simulink model "model"  (R2012b)
settings: Solver=ode45  StartTime=0.0  StopTime=10.0  MaxStep=0.2  RelTol=1e-3
settings Model: Creator=Vojta  LastModifiedBy=Pavilion
settings DataIOCC: SignalLoggingSaveFormat=ModelDataLogs
settings OptimizationCC: ExpressionDepthLimit=128
settings DebuggingCC: MultiTaskDSMMsg=warning  MultiTaskCondExecSysMsg=none  StateNameClashWarn=none  StrictBusMsg=None
settings RTWCC: IncludeERTFirstTime=on
settings CodeAppCC: CustomSymbolStrType=$N$R$M_T  InternalIdentifier=Shortened

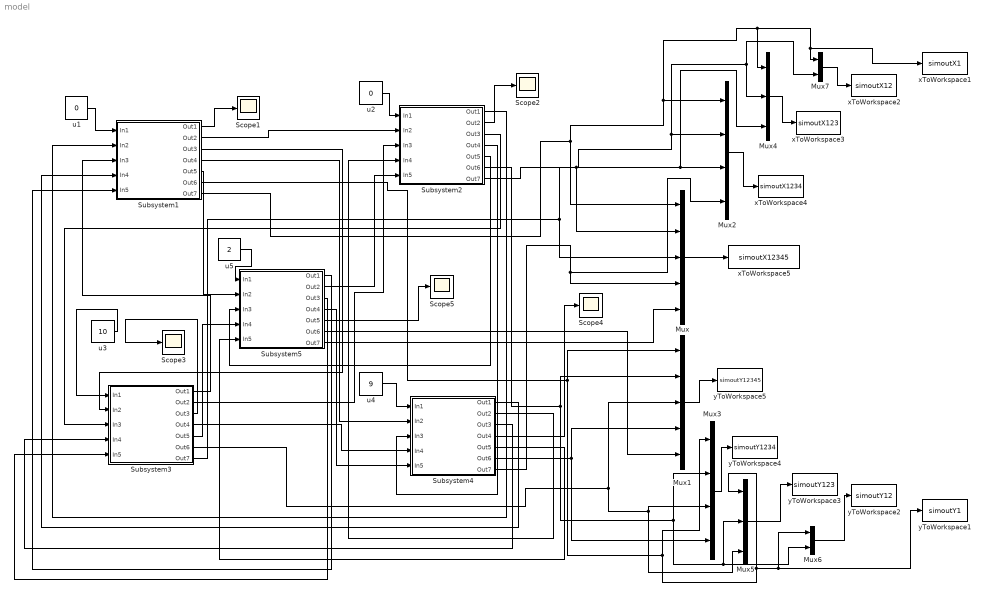
== system model ==
  Mux : Mux  Inputs=5
  Mux1 : Mux  Inputs=5
  Mux2 : Mux
  Mux3 : Mux
  Mux4 : Mux  Inputs=3
  Mux5 : Mux  Inputs=3
  Mux6 : Mux  Inputs=2
  Mux7 : Mux  Inputs=2
  Scope{1..5} (5 alike) : Scope
      Scope2 settings: SaveName=ScopeData2
      Scope3 settings: SaveName=ScopeData3
      Scope4 settings: SaveName=ScopeData4
      Scope5 settings: SaveName=ScopeData5
  Subsystem1 : Subsystem
  Subsystem2 : Subsystem
  Subsystem3 : Subsystem
  Subsystem4 : Subsystem
  Subsystem5 : Subsystem
  u1 : Constant  Value=0
  u2 : Constant  Value=0
  u3 : Constant  Value=10
  u4 : Constant  Value=9
  u5 : Constant  Value=2
  xToWorkspace1 : ToWorkspace  VariableName=simoutX1  SampleTime=-1  SaveFormat=Timeseries
  xToWorkspace2 : ToWorkspace  VariableName=simoutX12  SampleTime=-1  SaveFormat=Structure With Time
  xToWorkspace3 : ToWorkspace  VariableName=simoutX123  SampleTime=-1  SaveFormat=Structure With Time
  xToWorkspace4 : ToWorkspace  VariableName=simoutX1234  SampleTime=-1  SaveFormat=Structure With Time
  xToWorkspace5 : ToWorkspace  VariableName=simoutX12345  SampleTime=-1  SaveFormat=Structure With Time
  yToWorkspace1 : ToWorkspace  VariableName=simoutY1  SampleTime=-1  SaveFormat=Timeseries
  yToWorkspace2 : ToWorkspace  VariableName=simoutY12  SampleTime=-1  SaveFormat=Structure With Time
  yToWorkspace3 : ToWorkspace  VariableName=simoutY123  SampleTime=-1  SaveFormat=Structure With Time
  yToWorkspace4 : ToWorkspace  VariableName=simoutY1234  SampleTime=-1  SaveFormat=Structure With Time
  yToWorkspace5 : ToWorkspace  VariableName=simoutY12345  SampleTime=-1  SaveFormat=Structure With Time
  wires:
  u1/1 -> Subsystem1/1(In1)
  u2/1 -> Subsystem2/1(In1)
  u3/1 -> Subsystem3/1(In1)
  u4/1 -> Subsystem4/1(In1)
  u5/1 -> Subsystem5/1(In1)
  Subsystem1/7(Out7) -> xToWorkspace1/1, Mux7/1, Mux4/1, Mux2/1, Mux/1
  Subsystem2/7(Out7) -> Mux7/2, Mux4/2, Mux2/2, Mux/2
  Subsystem3/7(Out7) -> Mux4/3, Mux2/3, Mux/3
  Subsystem4/7(Out7) -> Mux/4, Mux2/4
  Subsystem1/6(Out6) -> yToWorkspace1/1, Mux6/1, Mux5/1, Mux3/1, Mux1/1
  Subsystem2/6(Out6) -> Mux6/2, Mux5/2, Mux3/2, Mux1/2
  Subsystem4/6(Out6) -> Mux3/4, Mux1/4
  Subsystem3/6(Out6) -> Mux1/3, Mux5/3, Mux3/3
  Mux/1 -> xToWorkspace5/1
  Mux1/1 -> yToWorkspace5/1
  Subsystem1/2(Out2) -> Subsystem2/2(In2)
  Subsystem1/3(Out3) -> Subsystem3/2(In2)
  Subsystem1/4(Out4) -> Subsystem4/2(In2)
  Subsystem1/5(Out5) -> Subsystem5/2(In2)
  Subsystem2/1(Out1) -> Subsystem1/2(In2)
  Subsystem2/3(Out3) -> Subsystem3/3(In3)
  Subsystem2/4(Out4) -> Subsystem4/3(In3)
  Subsystem2/5(Out5) -> Subsystem5/3(In3)
  Subsystem3/1(Out1) -> Subsystem1/3(In3)
  Subsystem3/2(Out2) -> Subsystem2/3(In3)
  Subsystem3/4(Out4) -> Subsystem4/4(In4)
  Subsystem3/5(Out5) -> Subsystem5/4(In4)
  Subsystem4/1(Out1) -> Subsystem1/4(In4)
  Subsystem4/2(Out2) -> Subsystem2/4(In4)
  Subsystem4/3(Out3) -> Subsystem3/4(In4)
  Subsystem4/5(Out5) -> Subsystem5/5(In5)
  Subsystem5/1(Out1) -> Subsystem1/5(In5)
  Subsystem5/2(Out2) -> Subsystem2/5(In5)
  Subsystem5/3(Out3) -> Subsystem3/5(In5)
  Subsystem5/4(Out4) -> Subsystem4/5(In5)
  Mux2/1 -> xToWorkspace4/1
  Mux4/1 -> xToWorkspace3/1
  Mux7/1 -> xToWorkspace2/1
  Mux3/1 -> yToWorkspace4/1
  Mux5/1 -> yToWorkspace3/1
  Mux6/1 -> yToWorkspace2/1
  Subsystem5/7(Out7) -> Mux/5
  Subsystem5/6(Out6) -> Mux1/5
  Subsystem1/1(Out1) -> Scope1/1
  Subsystem5/5(Out5) -> Scope5/1
  Subsystem4/4(Out4) -> Scope4/1
  Subsystem3/3(Out3) -> Scope3/1
  Subsystem2/2(Out2) -> Scope2/1

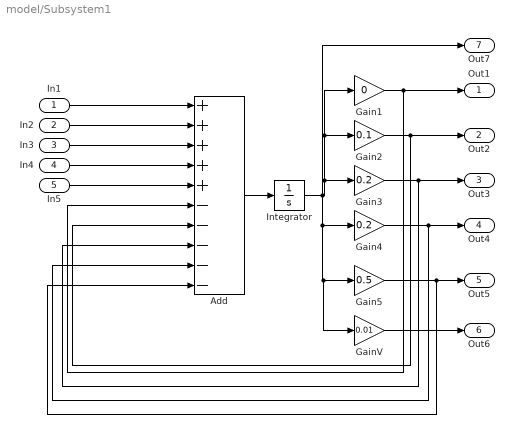
== system model/Subsystem1 ==
  In1 : Inport
  In2 : Inport  Port=2
  In3 : Inport  Port=3
  In4 : Inport  Port=4
  In5 : Inport  Port=5
  Add : Sum  Inputs=+++++-----
  Gain1 : Gain  Gain=0
  Gain2 : Gain  Gain=0.1
  Gain3 : Gain  Gain=0.2
  Gain4 : Gain  Gain=0.2
  Gain5 : Gain  Gain=0.5
  GainV : Gain  Gain=0.01
  Integrator : Integrator  InitialCondition=70
  Out1 : Outport
  Out2 : Outport  Port=2
  Out3 : Outport  Port=3
  Out4 : Outport  Port=4
  Out5 : Outport  Port=5
  Out6 : Outport  Port=6
  Out7 : Outport  Port=7
  wires:
  In1/1 -> Add/1
  In2/1 -> Add/2
  In3/1 -> Add/3
  In4/1 -> Add/4
  In5/1 -> Add/5
  Add/1 -> Integrator/1
  Integrator/1 -> Out7/1, GainV/1, Gain5/1, Gain4/1, Gain3/1, Gain2/1, Gain1/1
  Gain1/1 -> Add/6, Out1/1
  Gain2/1 -> Add/7, Out2/1
  Gain3/1 -> Add/8, Out3/1
  Gain4/1 -> Add/9, Out4/1
  Gain5/1 -> Add/10, Out5/1
  GainV/1 -> Out6/1

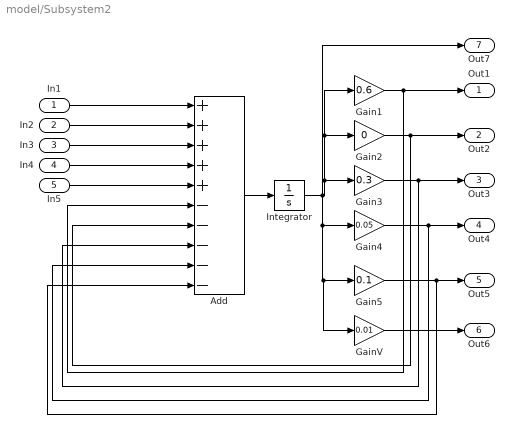
== system model/Subsystem2 ==
  In1 : Inport
  In2 : Inport  Port=2
  In3 : Inport  Port=3
  In4 : Inport  Port=4
  In5 : Inport  Port=5
  Add : Sum  Inputs=+++++-----
  Gain1 : Gain  Gain=0.6
  Gain2 : Gain  Gain=0
  Gain3 : Gain  Gain=0.3
  Gain4 : Gain  Gain=0.05
  Gain5 : Gain  Gain=0.1
  GainV : Gain  Gain=0.01
  Integrator : Integrator  InitialCondition=100
  Out1 : Outport
  Out2 : Outport  Port=2
  Out3 : Outport  Port=3
  Out4 : Outport  Port=4
  Out5 : Outport  Port=5
  Out6 : Outport  Port=6
  Out7 : Outport  Port=7
  wires:
  GainV/1 -> Out6/1
  Gain5/1 -> Out5/1, Add/10
  Gain4/1 -> Out4/1, Add/9
  Gain3/1 -> Out3/1, Add/8
  Gain2/1 -> Out2/1, Add/7
  Gain1/1 -> Out1/1, Add/6
  Integrator/1 -> Gain1/1, Gain2/1, Gain3/1, Gain4/1, Gain5/1, GainV/1, Out7/1
  Add/1 -> Integrator/1
  In5/1 -> Add/5
  In4/1 -> Add/4
  In3/1 -> Add/3
  In2/1 -> Add/2
  In1/1 -> Add/1

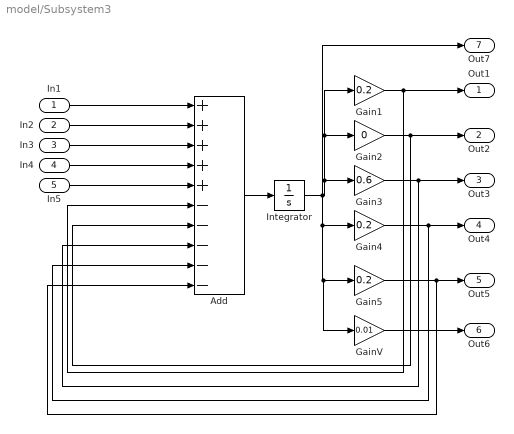
== system model/Subsystem3 ==
  In1 : Inport
  In2 : Inport  Port=2
  In3 : Inport  Port=3
  In4 : Inport  Port=4
  In5 : Inport  Port=5
  Add : Sum  Inputs=+++++-----
  Gain1 : Gain  Gain=0.2
  Gain2 : Gain  Gain=0
  Gain3 : Gain  Gain=0.6
  Gain4 : Gain  Gain=0.2
  Gain5 : Gain  Gain=0.2
  GainV : Gain  Gain=0.01
  Integrator : Integrator  InitialCondition=70
  Out1 : Outport
  Out2 : Outport  Port=2
  Out3 : Outport  Port=3
  Out4 : Outport  Port=4
  Out5 : Outport  Port=5
  Out6 : Outport  Port=6
  Out7 : Outport  Port=7
  wires:
  GainV/1 -> Out6/1
  Gain5/1 -> Out5/1, Add/10
  Gain4/1 -> Out4/1, Add/9
  Gain3/1 -> Out3/1, Add/8
  Gain2/1 -> Out2/1, Add/7
  Gain1/1 -> Out1/1, Add/6
  Integrator/1 -> Gain1/1, Gain2/1, Gain3/1, Gain4/1, Gain5/1, GainV/1, Out7/1
  Add/1 -> Integrator/1
  In5/1 -> Add/5
  In4/1 -> Add/4
  In3/1 -> Add/3
  In2/1 -> Add/2
  In1/1 -> Add/1

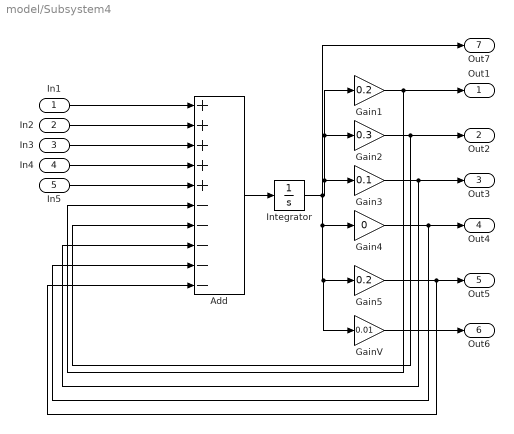
== system model/Subsystem4 ==
  In1 : Inport
  In2 : Inport  Port=2
  In3 : Inport  Port=3
  In4 : Inport  Port=4
  In5 : Inport  Port=5
  Add : Sum  Inputs=+++++-----
  Gain1 : Gain  Gain=0.2
  Gain2 : Gain  Gain=0.3
  Gain3 : Gain  Gain=0.1
  Gain4 : Gain  Gain=0
  Gain5 : Gain  Gain=0.2
  GainV : Gain  Gain=0.01
  Integrator : Integrator
  Out1 : Outport
  Out2 : Outport  Port=2
  Out3 : Outport  Port=3
  Out4 : Outport  Port=4
  Out5 : Outport  Port=5
  Out6 : Outport  Port=6
  Out7 : Outport  Port=7
  wires:
  In1/1 -> Add/1
  In2/1 -> Add/2
  In3/1 -> Add/3
  In4/1 -> Add/4
  In5/1 -> Add/5
  Add/1 -> Integrator/1
  Integrator/1 -> Out7/1, GainV/1, Gain5/1, Gain4/1, Gain3/1, Gain2/1, Gain1/1
  Gain1/1 -> Add/6, Out1/1
  Gain2/1 -> Add/7, Out2/1
  Gain3/1 -> Add/8, Out3/1
  Gain4/1 -> Add/9, Out4/1
  Gain5/1 -> Add/10, Out5/1
  GainV/1 -> Out6/1

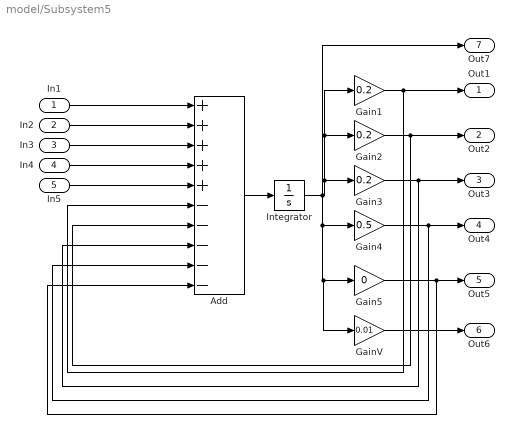
== system model/Subsystem5 ==
  In1 : Inport
  In2 : Inport  Port=2
  In3 : Inport  Port=3
  In4 : Inport  Port=4
  In5 : Inport  Port=5
  Add : Sum  Inputs=+++++-----
  Gain1 : Gain  Gain=0.2
  Gain2 : Gain  Gain=0.2
  Gain3 : Gain  Gain=0.2
  Gain4 : Gain  Gain=0.5
  Gain5 : Gain  Gain=0
  GainV : Gain  Gain=0.01
  Integrator : Integrator
  Out1 : Outport
  Out2 : Outport  Port=2
  Out3 : Outport  Port=3
  Out4 : Outport  Port=4
  Out5 : Outport  Port=5
  Out6 : Outport  Port=6
  Out7 : Outport  Port=7
  wires:
  GainV/1 -> Out6/1
  Gain5/1 -> Out5/1, Add/10
  Gain4/1 -> Out4/1, Add/9
  Gain3/1 -> Out3/1, Add/8
  Gain2/1 -> Out2/1, Add/7
  Gain1/1 -> Out1/1, Add/6
  Integrator/1 -> Gain1/1, Gain2/1, Gain3/1, Gain4/1, Gain5/1, GainV/1, Out7/1
  Add/1 -> Integrator/1
  In5/1 -> Add/5
  In4/1 -> Add/4
  In3/1 -> Add/3
  In2/1 -> Add/2
  In1/1 -> Add/1
